simulink model "Modello_carroponte_lineare"  (R2024a)
settings: Solver=VariableStepAuto  StartTime=tempo(1)  StopTime=tempo(end)  FixedStep=dt  RelTol=1e-3
undefined symbols (not defined in the file): alpha_0_eq, alpha_dot_0_eq, cc, cm, dinamica_alpha, g, L, mc, mm, xc_0_eq, xc_dot_0_eq
libraries: simulink x1
settings Model: Creator=smila  LastModifiedBy=smila
settings OptimizationCC: BlockReduction=off  DefaultParameterBehavior=Inlined  BufferReuse=off

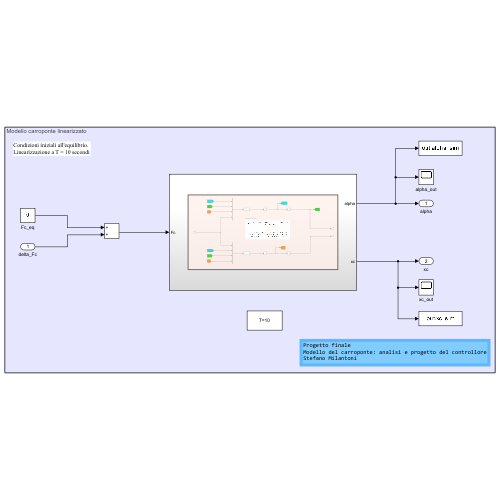
[thumbnail: Simulink's stored preview of the top-level diagram]
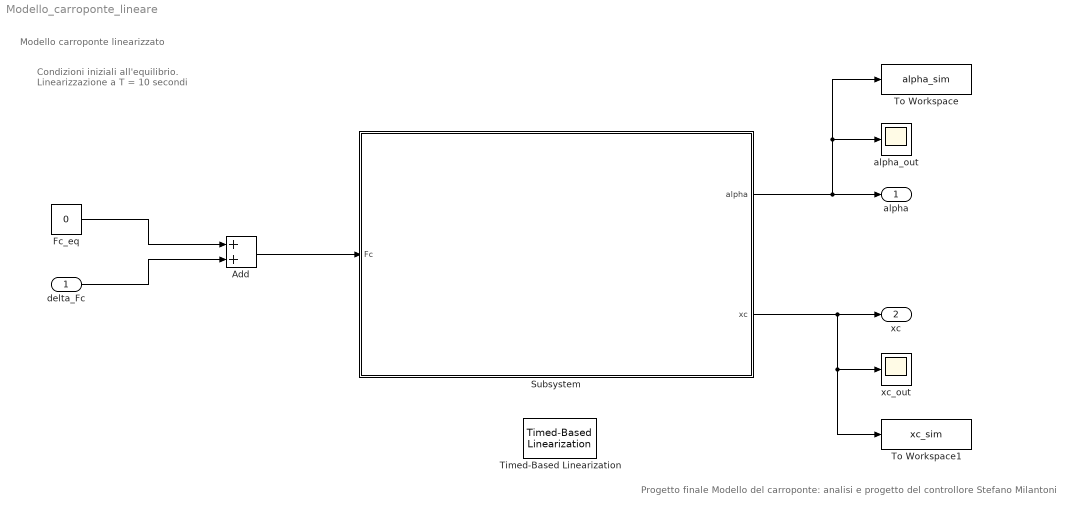
== system Modello_carroponte_lineare ==
  note: Condizioni iniziali all'equilibrio.
      | Linearizzazione a T = 10 secondi
  note: Modello carroponte linearizzato
  note: Progetto finale
      | Modello del carroponte: analisi e progetto del controllore
      | Stefano Milantoni
  delta_Fc : Inport
  Add : Sum
  Fc_eq : Constant  Value=0
  Subsystem : Subsystem
  Timed-Based Linearization : simulink/Model-Wide Utilities/Timed-Based Linearization  LinearizationTime=10  SampleTime=0
  To Workspace : ToWorkspace  VariableName=alpha_sim  SampleTime=-1
  To Workspace1 : ToWorkspace  VariableName=xc_sim  SampleTime=-1
  alpha_out : Scope
  xc_out : Scope
  alpha : Outport
  xc : Outport  Port=2
  wires:
  Add/1 -> Subsystem/1(Fc)
  Fc_eq/1 -> Add/1
  delta_Fc/1 -> Add/2
  Subsystem/1(alpha) -> alpha_out/1, To Workspace/1, alpha/1
  Subsystem/2(xc) -> To Workspace1/1, xc_out/1, xc/1

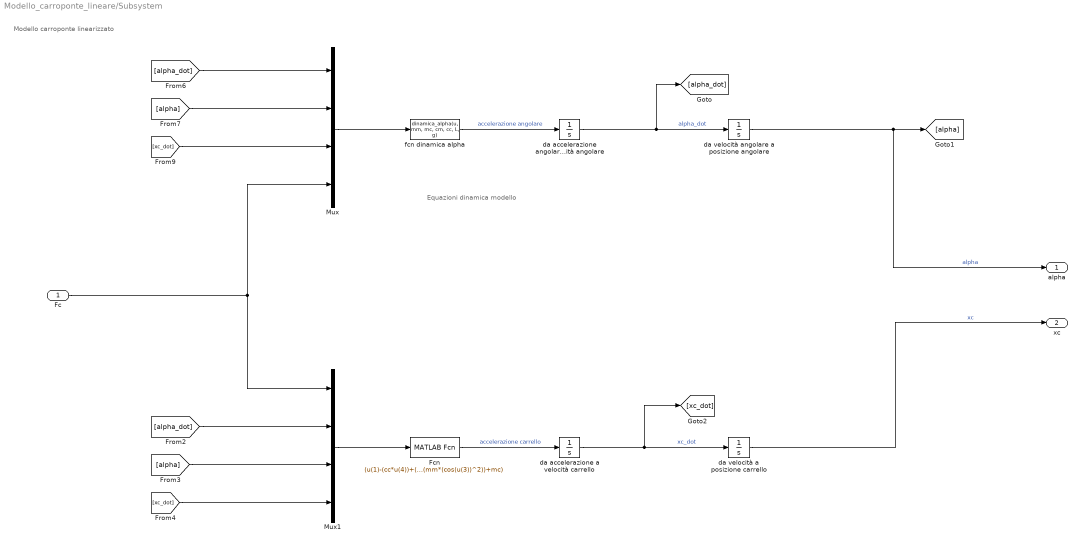
== system Modello_carroponte_lineare/Subsystem ==
  note: Equazioni dinamica modello
  note: Modello carroponte linearizzato
  Fc : Inport
  Fcn : MATLABFcn  MATLABFcn=(u(1)-(cc*u(4))+(mm*g*sin(u(3))*cos(u(3)))-(cm*u(4)*(cos(u(3))^2))+(mm*L*cos(u(3))*(u(2)^2)))/((mm*(cos(u(3))^2))+mc)
  Mux : Mux
  Mux1 : Mux
  da accelerazione a velocità carrello : Integrator  InitialCondition=xc_dot_0_eq
  da accelerazione angolare a velocità angolare : Integrator  InitialCondition=alpha_dot_0_eq
  da velocità a posizione carrello : Integrator  InitialCondition=xc_0_eq
  da velocità angolare a posizione angolare : Integrator  InitialCondition=alpha_0_eq
  fcn dinamica alpha : MATLABFcn  MATLABFcn=dinamica_alpha(u, mm, mc, cm, cc, L, g)
  alpha : Outport
  xc : Outport  Port=2
  wires:
  da accelerazione a velocità carrello/1 -> da velocità a posizione carrello/1, [xc_dot]  "xc_dot"
  da velocità a posizione carrello/1 -> xc/1  "xc"
  da accelerazione angolare a velocità angolare/1 -> da velocità angolare a posizione angolare/1, [alpha_dot]  "alpha_dot"
  Mux1/1 -> Fcn/1
  [xc_dot] -> Mux1/4
  Mux/1 -> fcn dinamica alpha/1
  Fcn/1 -> da accelerazione a velocità carrello/1  "accelerazione carrello"
  Fc/1 -> Mux1/1, Mux/4
  fcn dinamica alpha/1 -> da accelerazione angolare a velocità angolare/1  "accelerazione angolare"
  da velocità angolare a posizione angolare/1 -> alpha/1, [alpha]  "alpha"
  [alpha_dot] -> Mux1/2
  [alpha] -> Mux1/3
  [alpha_dot] -> Mux/1
  [alpha] -> Mux/2
  [xc_dot] -> Mux/3
